simulink model "acdcmg_sim8_2_sc_gui"  (R2019b)
settings: Solver=ode8  StartTime=0.0  StopTime=0.5  FixedStep=4e-05  MaxStep=1e-2  RelTol=1e-3
PreLoadFcn:
  | Set_parameters_R2018
InitFcn:
  | Set_parameters_R2018
libraries: opal_lib x23
(part 2 of 2)

== system acdcmg_sim8_2_sc_gui/OpComm2/busStruct/Sub1 ==
  in : Inport
  out : Outport
  wires:
  in/1 -> out/1  "signal1"

== system acdcmg_sim8_2_sc_gui/OpComm2/busStruct/Sub2 ==
  in : Inport
  out : Outport
  wires:
  in/1 -> out/1  "signal1"

== system acdcmg_sim8_2_sc_gui/OpComm2/busStruct/Sub3 ==
  in : Inport
  out : Outport
  wires:
  in/1 -> out/1  "signal"

== system acdcmg_sim8_2_sc_gui/OpComm2/busStruct/Sub4 ==
  in : Inport
  out : Outport
  wires:
  in/1 -> out/1  "signal1"

== system acdcmg_sim8_2_sc_gui/OpComm20/busStruct/Sub1 ==
  in : Inport
  out : Outport
  wires:
  in/1 -> out/1  "signal1"

== system acdcmg_sim8_2_sc_gui/OpComm20/busStruct/Sub2 ==
  in : Inport
  out : Outport
  wires:
  in/1 -> out/1  "signal1"

== system acdcmg_sim8_2_sc_gui/OpComm20/busStruct/Sub3 ==
  in : Inport
  out : Outport
  wires:
  in/1 -> out/1  "signal1"

== system acdcmg_sim8_2_sc_gui/OpComm20/busStruct/Sub4 ==
  in : Inport
  out : Outport
  wires:
  in/1 -> out/1  "signal1"

== system acdcmg_sim8_2_sc_gui/OpComm21/busStruct/Sub1 ==
  in : Inport
  out : Outport
  wires:
  in/1 -> out/1  "signal1"

== system acdcmg_sim8_2_sc_gui/OpComm21/busStruct/Sub2 ==
  in : Inport
  out : Outport
  wires:
  in/1 -> out/1  "signal1"

== system acdcmg_sim8_2_sc_gui/OpComm3/busStruct/Sub1 ==
  in : Inport
  out : Outport
  wires:
  in/1 -> out/1  "D_Pa_kW"

== system acdcmg_sim8_2_sc_gui/OpComm3/busStruct/Sub2 ==
  in : Inport
  out : Outport
  wires:
  in/1 -> out/1  "D_Pb_kW"

== system acdcmg_sim8_2_sc_gui/OpComm3/busStruct/Sub3 ==
  in : Inport
  out : Outport
  wires:
  in/1 -> out/1  "D_Pc_kW"

== system acdcmg_sim8_2_sc_gui/OpComm3/busStruct/Sub4 ==
  in : Inport
  out : Outport
  wires:
  in/1 -> out/1  "signal1"

== system acdcmg_sim8_2_sc_gui/OpComm4/busStruct/Sub1 ==
  in : Inport
  out : Outport
  wires:
  in/1 -> out/1  "signal1"

== system acdcmg_sim8_2_sc_gui/OpComm4/busStruct/Sub2 ==
  in : Inport
  out : Outport
  wires:
  in/1 -> out/1  "signal1"

== system acdcmg_sim8_2_sc_gui/OpComm4/busStruct/Sub3 ==
  in : Inport
  out : Outport
  wires:
  in/1 -> out/1  "signal1"

== system acdcmg_sim8_2_sc_gui/OpComm4/busStruct/Sub4 ==
  in : Inport
  out : Outport
  wires:
  in/1 -> out/1  "signal"

== system acdcmg_sim8_2_sc_gui/OpComm5/busStruct/Sub1 ==
  in : Inport
  out : Outport
  wires:
  in/1 -> out/1  "D_Pa_kW"

== system acdcmg_sim8_2_sc_gui/OpComm5/busStruct/Sub2 ==
  in : Inport
  out : Outport
  wires:
  in/1 -> out/1  "D_Pb_kW"

== system acdcmg_sim8_2_sc_gui/OpComm5/busStruct/Sub3 ==
  in : Inport
  out : Outport
  wires:
  in/1 -> out/1  "D_Pc_kW"

== system acdcmg_sim8_2_sc_gui/OpComm5/busStruct/Sub4 ==
  in : Inport
  out : Outport
  wires:
  in/1 -> out/1  "signal1"

== system acdcmg_sim8_2_sc_gui/OpComm6/busStruct/Sub1 ==
  in : Inport
  out : Outport
  wires:
  in/1 -> out/1  "D_Pa_kW"

== system acdcmg_sim8_2_sc_gui/OpComm6/busStruct/Sub2 ==
  in : Inport
  out : Outport
  wires:
  in/1 -> out/1  "D_Pb_kW"

== system acdcmg_sim8_2_sc_gui/OpComm6/busStruct/Sub3 ==
  in : Inport
  out : Outport
  wires:
  in/1 -> out/1  "D_Pc_kW"

== system acdcmg_sim8_2_sc_gui/OpComm6/busStruct/Sub4 ==
  in : Inport
  out : Outport
  wires:
  in/1 -> out/1  "signal1"

== system acdcmg_sim8_2_sc_gui/OpComm7/busStruct/Sub1 ==
  in : Inport
  out : Outport
  wires:
  in/1 -> out/1  "D_Pa_kW"

== system acdcmg_sim8_2_sc_gui/OpComm7/busStruct/Sub2 ==
  in : Inport
  out : Outport
  wires:
  in/1 -> out/1  "D_Pb_kW"

== system acdcmg_sim8_2_sc_gui/OpComm7/busStruct/Sub3 ==
  in : Inport
  out : Outport
  wires:
  in/1 -> out/1  "D_Pc_kW"

== system acdcmg_sim8_2_sc_gui/OpComm7/busStruct/Sub4 ==
  in : Inport
  out : Outport
  wires:
  in/1 -> out/1  "signal1"

== system acdcmg_sim8_2_sc_gui/OpComm8/busStruct/Sub1 ==
  in : Inport
  out : Outport
  wires:
  in/1 -> out/1  "signal1"

== system acdcmg_sim8_2_sc_gui/OpComm8/busStruct/Sub2 ==
  in : Inport
  out : Outport
  wires:
  in/1 -> out/1  "signal1"

== system acdcmg_sim8_2_sc_gui/OpComm8/busStruct/Sub3 ==
  in : Inport
  out : Outport
  wires:
  in/1 -> out/1  "signal1"

== system acdcmg_sim8_2_sc_gui/OpComm8/busStruct/Sub4 ==
  in : Inport
  out : Outport
  wires:
  in/1 -> out/1  "signal"

== system acdcmg_sim8_2_sc_gui/OpComm9/busStruct/Sub1 ==
  in : Inport
  out : Outport
  wires:
  in/1 -> out/1  "signal1"

== system acdcmg_sim8_2_sc_gui/OpComm9/busStruct/Sub2 ==
  in : Inport
  out : Outport
  wires:
  in/1 -> out/1  "signal1"

== system acdcmg_sim8_2_sc_gui/OpComm9/busStruct/Sub3 ==
  in : Inport
  out : Outport
  wires:
  in/1 -> out/1  "signal1"

== system acdcmg_sim8_2_sc_gui/OpComm9/busStruct/Sub4 ==
  in : Inport
  out : Outport
  wires:
  in/1 -> out/1  "signal"
